simulink model "Design_of_Three_Phase_Transformer"  (R2025a)
settings: Solver=ode23tb  StartTime=0.0  StopTime=0.2  MaxStep=1e-4  RelTol=1e-3
libraries: spsRMSLib x4, spsACVoltageSourceLib x3, spsThreePhaseVIMeasurementLib x2, spsGroundLib x1, spsThreePhaseSeriesRLCLoadLib x1, spsThreePhaseTransformerTwoWindingsLib x1, sps_lib x1
settings Model: Creator=Jawad  LastModifiedBy=Jawad

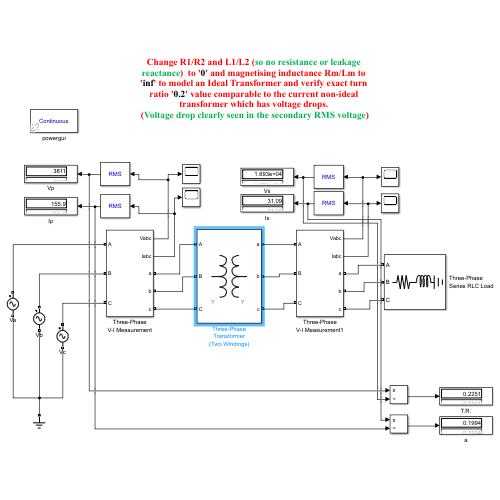
[thumbnail: Simulink's stored preview of the top-level diagram]
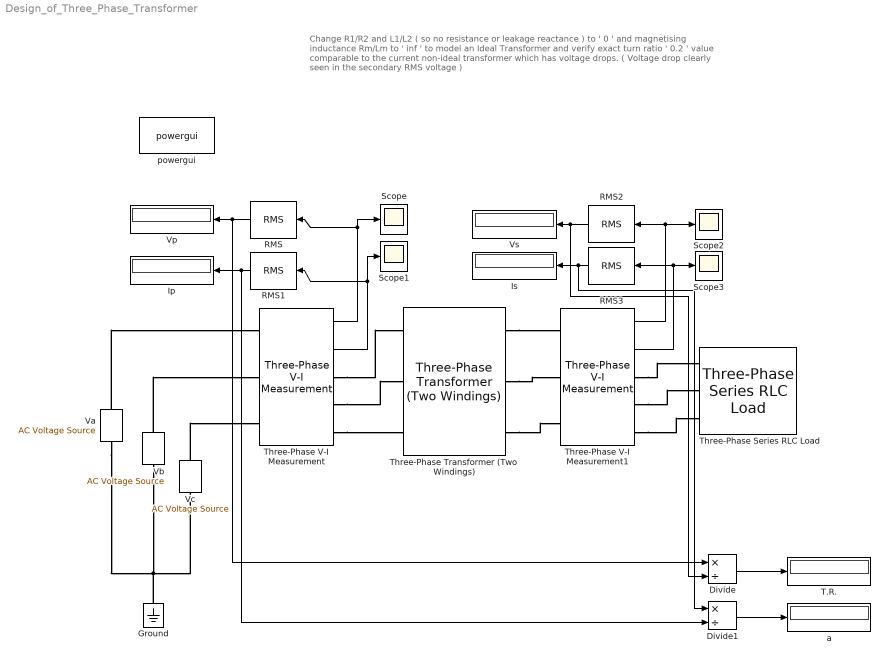
== system Design_of_Three_Phase_Transformer ==
  note: Change R1/R2 and L1/L2 ( so no resistance or leakage reactance ) to ' 0 ' and magnetising inductance Rm/Lm to ' inf ' to model an Ideal Transformer and verify exact turn ratio ' 0.2 ' value comparable to the current non-ideal transformer which has voltage drops.
      | ( Voltage drop clearly seen in the secondary RMS voltage )
  Divide : Product  Inputs=*/
  Divide1 : Product  Inputs=*/
  Ground : spsGroundLib/Ground  LConnTagsString=a
  Ip : Display
  Is : Display
  RMS{,1..3} (4 alike) : spsRMSLib/RMS  TrueRMS=off  Freq=50  RMSInit=0  Ts=0
  Scope{,1..3} (4 alike) : Scope
      Scope settings: ActiveDisplayYMinimum=-6736.0902871668777  ActiveDisplayYMaximum=6736.0893810743028
      Scope2 settings: DataLoggingVariableName=ScopeData2
      Scope3 settings: ActiveDisplayYMinimum=-1  ActiveDisplayYMaximum=1  DataLoggingVariableName=ScopeData3
  T.R. : Display
  Three-Phase Series RLC Load : spsThreePhaseSeriesRLCLoadLib/Three-Phase Series RLC Load  LConnTagsString=A|B|C  Configuration=Y (grounded)  NominalVoltage=33e3  Vabc=[1e3 1e3 1e3]  Vabcp=[1e3 1e3 1e3]  NominalFrequency=50  UnbalancedPower=off  ActivePower=1600e3  InductivePower=1200e3  CapacitivePower=0  Pabc=[10e3 9e3 11e3]  QLabc=[100 90 110]  QCabc=[100 90 110]  Pabcp=[10e3 9e3 11e3]  QLabcp=[100 90 110]  QCabcp=[100 90 110]  Measurements=None  LoadType=constant Z
  Three-Phase Transformer (Two Windings) : spsThreePhaseTransformerTwoWindingsLib/Three-Phase Transformer (Two Windings)  Winding1Connection=Y  Winding2Connection=Y  CoreType=Three single-phase transformers  SetSaturation=off  Hysteresis=off  DataFile='hysteresis'  SetInitialFlux=off  Measurements=None  UNITS=SI  NominalPower=[ 200e3 , 50 ]  Winding1=[6600 0.5 8.27e-3]  Winding2=[33e3 4.3 0.069]  Rm=10890  Lm=34.664  L0=0.28887  Saturation=[0 0;0.059382 17.153;24.742 21.728]  InitialFluxes=[11.436 -11.436 10.006]  BreakLoop=off  DiscreteSolver=Trapezoidal iterative  DataType=on  TransfoNumber=1
  Three-Phase V-I Measurement : spsThreePhaseVIMeasurementLib/Three-Phase V-I Measurement  VoltageMeasurement=phase-to-ground  SetLabelV=off  LabelV=Vabc  Vpu=off  VpuLL=off  CurrentMeasurement=yes  SetLabelI=off  LabelI=Iabc  Ipu=off  Pbase=100e6  Vbase=500e3  OutputType=Complex  PhasorSimulation=off  PSBequivalent=0
  Three-Phase V-I Measurement1 : spsThreePhaseVIMeasurementLib/Three-Phase V-I Measurement  VoltageMeasurement=phase-to-ground  SetLabelV=off  LabelV=Vabc  Vpu=off  VpuLL=off  CurrentMeasurement=yes  SetLabelI=off  LabelI=Iabc  Ipu=off  Pbase=100e6  Vbase=500e3  OutputType=Complex  PhasorSimulation=off  PSBequivalent=0
  Va : spsACVoltageSourceLib/AC Voltage Source  Amplitude=(6.6e3*sqrt(2))/sqrt(3)  Phase=0  Frequency=50  SampleTime=0  Measurements=None  BusType=swing  Pref=10e3  Qref=0  Qmin=-inf  Qmax=+inf
  Vb : spsACVoltageSourceLib/AC Voltage Source  Amplitude=(6.6e3*sqrt(2))/sqrt(3)  Phase=-120  Frequency=50  SampleTime=0  Measurements=None  BusType=swing  Pref=10e3  Qref=0  Qmin=-inf  Qmax=+inf
  Vc : spsACVoltageSourceLib/AC Voltage Source  Amplitude=(6.6e3*sqrt(2))/sqrt(3)  Phase=120  Frequency=50  SampleTime=0  Measurements=None  BusType=swing  Pref=10e3  Qref=0  Qmin=-inf  Qmax=+inf
  Vp : Display
  Vs : Display
  a : Display
  powergui : sps_lib/powergui  Priority=1  SimulationMode=Continuous  SampleTime=50e-6  frequency=60  Iterations=50  frequencyindice=50  Pbase=100e6  ErrMax=1e-4  UnitsV=kV  UnitsW=MW  buscounter=0  FunctionMessages=off  echomessages=off  EnableUseOfTLC=off  CurrentSourceSwitches=off  DisableSnubberDevices=off  DisableRonSwitches=off  DisableVfSwitches=off  DisplayEquations=off  AutomaticDiscreteSolvers=off  SolverType=Tustin/Backward Euler (TBE)  Interpol=off  ExternalGateDelay=off  methode=off  Ts=100  x0status=blocks  SPID=on  SwTol=0  HookPort=off  NonlinearTolerance=1e-4  nMaxIteration=100  ContinueOnMaxIteration=off  RestoreLinks=warning  ResistiveCurrentMeasurement=off  Frange=[0:2:500]  Ylog=off  Xlog=on  ShowGrid=off  save=off  variable=ZData  structure=0  ZoomFFT=off  StartTime=0.0  cycles=1  DisplayStyle=1  fundamental=60  FreqAxis=off  MaxFrequency=1000  frequencyindicesteady=1  RmsSteady=1  display=off
  wires:
  Three-Phase V-I Measurement/1 -> Scope/1, RMS/1
  Three-Phase V-I Measurement/2 -> Scope1/1, RMS1/1
  RMS/1 -> Divide/1, Vp/1
  RMS1/1 -> Divide1/2, Ip/1
  Three-Phase V-I Measurement1/1 -> Scope2/1, RMS2/1
  Three-Phase V-I Measurement1/2 -> Scope3/1, RMS3/1
  RMS2/1 -> Divide/2, Vs/1
  RMS3/1 -> Divide1/1, Is/1
  Divide/1 -> T.R./1
  Divide1/1 -> a/1
  connections:
  Va/LConn1 -- Ground/LConn1 -- Vb/LConn1 -- Vc/LConn1
  Vc/RConn1 -- Three-Phase V-I Measurement/LConn3
  Vb/RConn1 -- Three-Phase V-I Measurement/LConn2
  Va/RConn1 -- Three-Phase V-I Measurement/LConn1
  Three-Phase V-I Measurement/RConn1 -- Three-Phase Transformer (Two Windings)/LConn1
  Three-Phase V-I Measurement/RConn2 -- Three-Phase Transformer (Two Windings)/LConn2
  Three-Phase V-I Measurement/RConn3 -- Three-Phase Transformer (Two Windings)/LConn3
  Three-Phase Transformer (Two Windings)/RConn1 -- Three-Phase V-I Measurement1/LConn1
  Three-Phase Transformer (Two Windings)/RConn2 -- Three-Phase V-I Measurement1/LConn2
  Three-Phase Transformer (Two Windings)/RConn3 -- Three-Phase V-I Measurement1/LConn3
  Three-Phase V-I Measurement1/RConn1 -- Three-Phase Series RLC Load/LConn1
  Three-Phase V-I Measurement1/RConn2 -- Three-Phase Series RLC Load/LConn2
  Three-Phase V-I Measurement1/RConn3 -- Three-Phase Series RLC Load/LConn3
